simulink model "DSB_TC_Receiver_Part_2_2"  (R2022a)
settings: Solver=FixedStepDiscrete  StartTime=0.0  StopTime=inf  RelTol=1e-3
PreLoadFcn:
  | addpath('matlab/DSB_TC');
libraries: matrix_library x2, dspsnks4 x1, dspvision x1, dspstat3 x1, dspsigops x1
settings Model: Creator=vovan  LastModifiedBy=vovan

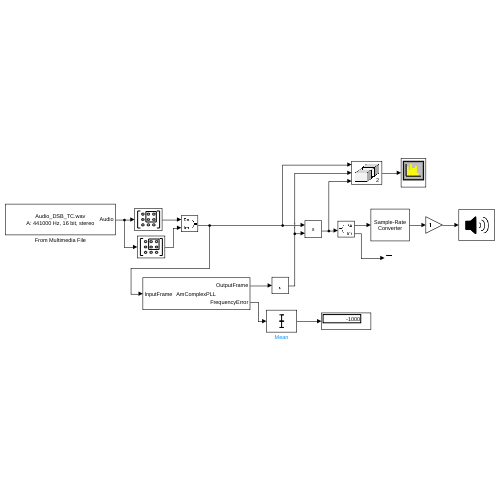
[thumbnail: Simulink's stored preview of the top-level diagram]
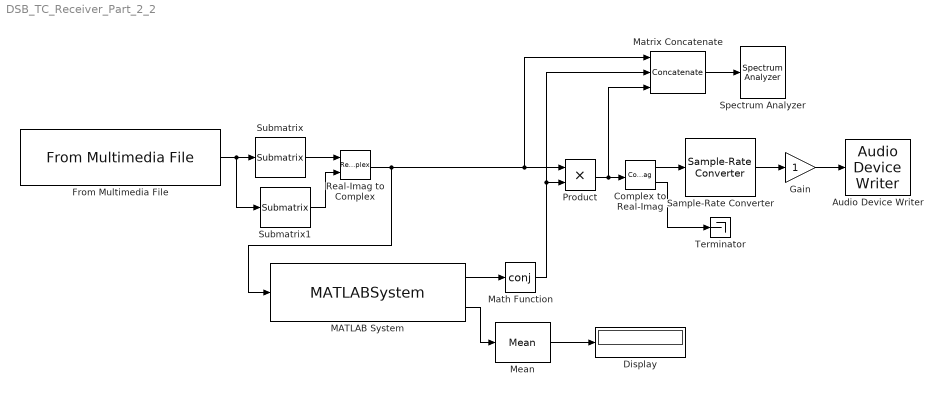
== system DSB_TC_Receiver_Part_2_2 ==
  Audio Device Writer : dspsnks4/Audio Device Writer  Driver=ALSA  Device=Default  InheritSampleRate=on  SampleRate=44100  BitDepth=16-bit integer  BufferSize=4096  NumBuffers=10  DefaultOutputChannelMapping=on  OutputChannelMapping=1:2  OutputNumUnderrunSamples=off  DriverIdx=8  DeviceWarnFlag=''
  Complex to Real-Imag : ComplexToRealImag
  Display : Display
  From Multimedia File : dspvision/From Multimedia File  inputFilename=wav/Audio_DSB_TC.wav  readRange=[1 Inf]  loop=on  numPlays=inf  outputStreams=Audio only  videoDataType=single  audioDataType=double  inheritSampleTime=on  userDefinedSampleTime=1/30  noAudioOutput=off  isIntensityVideo=off  fourcc=RGB  colorVideoFormat=Separate color signals  outputEOF=off  dataOrg=Column-major  audioFrameSize=10000  computeAudioFrameSize=off  outSamplingMode=Sample based
  Gain : Gain
  MATLAB System : MATLABSystem  System=AmComplexPLL  SampleFrequency=441000  NoiseBandwidth=100  Dampingfactor=0.7  CentralFrequency=60e3 + 1000  SimulateUsing=Code generation
      mask Type: AmComplexPLL
      mask Display:
      | disp('AmComplexPLL');
      | port_label('input',1,'InputFrame');
      | port_label('output',1,'OutputFrame');
      | port_label('output',2,'FrequencyError');
  Math Function : Math  Operator=conj
  Matrix Concatenate : Concatenate  NumInputs=3  Mode=Multidimensional array  ConcatenateDimension=2
  Mean : dspstat3/Mean  run=off  InputProcessing=Columns as channels (frame based)  reset_popup=None  directionMode=Each column  dimension=1  roiEnable=off  roiType=Rectangles  roiPortion=Entire ROI  roiOutput=Individual statistics for each ROI  roiFlag=off  roundingMode=Floor  overflowMode=off  outputDataTypeStr=Inherit: Same as accumulator  outputMin=[]  outputMax=[]  outputLastDataTypeStr=Inherit: Same as accumulator
  Product : Product
  Real-Imag to Complex : RealImagToComplex
  Sample-Rate Converter : dspsigops/Sample-Rate Converter  InputSampleRate=441000  OutputSampleRate=44100  OutputRateTolerance=0  Bandwidth=40e3  StopbandAttenuation=80  SimulateUsing=Code generation
      settings: SourceProductBaseCode=DS
  Spectrum Analyzer : SpectrumAnalyzer
  Submatrix : matrix_library/Submatrix  RowSpan=All rows  RowStartMode=First  RowStartIndex=1  RowEndMode=Last  RowEndIndex=1  ColSpan=Range of columns  ColStartMode=First  ColStartIndex=1  ColEndMode=Index  ColEndIndex=1
      settings: SourceProductBaseCode=SL
  Submatrix1 : matrix_library/Submatrix  RowSpan=All rows  RowStartMode=First  RowStartIndex=1  RowEndMode=Last  RowEndIndex=1  ColSpan=Range of columns  ColStartMode=Last  ColStartIndex=1  ColEndMode=Index  ColEndIndex=1
      settings: SourceProductBaseCode=SL
  Terminator : Terminator
  wires:
  From Multimedia File/1 -> Submatrix1/1, Submatrix/1
  MATLAB System/1 -> Math Function/1
  Submatrix/1 -> Real-Imag to Complex/1
  Submatrix1/1 -> Real-Imag to Complex/2
  Real-Imag to Complex/1 -> Matrix Concatenate/1, Product/1, MATLAB System/1
  Complex to Real-Imag/2 -> Terminator/1
  Product/1 -> Matrix Concatenate/3, Complex to Real-Imag/1
  Sample-Rate Converter/1 -> Gain/1
  Complex to Real-Imag/1 -> Sample-Rate Converter/1
  Gain/1 -> Audio Device Writer/1
  Matrix Concatenate/1 -> Spectrum Analyzer/1
  Math Function/1 -> Matrix Concatenate/2, Product/2
  MATLAB System/2 -> Mean/1
  Mean/1 -> Display/1
